simulink model "exampleModel_bus_axi_lcls2"  (R2017b)
settings: Solver=VariableStepAuto  StartTime=0.0  StopTime=10e-5  RelTol=1e-3
PreLoadFcn:
  | setup
values from neighbouring files (symbols this model uses):
  axiClk = 156.25e6    (= 156250000)    [setup.m]    (also in setup_exampleModel_bus_axi_simulink.m; setup_exampleModel_bus_axi_simulink_lcls2.m; setup_lcls2_pcav.m; sysgen_signal.m)
  cav1p1_addr = 204    [setup_exampleModel_bus_axi_simulink.m]    (also in setup_exampleModel_bus_axi_simulink_lcls2.m; setup_lcls2_pcav.m; sysgen_signal.m)
  cav1p2_addr = cav1p1_addr * 2    (= 408)    [setup_exampleModel_bus_axi_simulink.m]    (also in setup_exampleModel_bus_axi_simulink_lcls2.m; setup_lcls2_pcav.m; sysgen_signal.m)
  cav2p1_addr = cav1p1_addr * 3    (= 612)    [setup_exampleModel_bus_axi_simulink.m]    (also in setup_exampleModel_bus_axi_simulink_lcls2.m; setup_lcls2_pcav.m; sysgen_signal.m)
  cav2p2_addr = cav1p1_addr * 4    (= 816)    [setup_exampleModel_bus_axi_simulink.m]    (also in setup_exampleModel_bus_axi_simulink_lcls2.m; setup_lcls2_pcav.m; sysgen_signal.m)
  Fadc = Fs/interleavedChannels    (= 29750000)    [setup.m]    (also in setup_exampleModel_bus_axi_simulink.m = 357000000; setup_exampleModel_bus_axi_simulink_lcls2.m = 351000000; setup_lcls2_pcav.m = 357000000; sysgen_signal.m = 357000000)
  Fproc = 204e6    (= 204000000)    [setup_exampleModel_bus_axi_simulink.m]    (also in setup_exampleModel_bus_axi_simulink_lcls2.m = 200571400; setup_lcls2_pcav.m; sysgen_signal.m)
  Fsig = Fproc/12    (= 17000000)    [setup_exampleModel_bus_axi_simulink.m]    (also in setup_exampleModel_bus_axi_simulink_lcls2.m = 16714283.3333; setup_lcls2_pcav.m)
  Tadc = 1/fadc    (= 2.80112044818e-09)    [cavity_signal.m]    (also in setup_exampleModel_bus_axi_simulink.m; setup_exampleModel_bus_axi_simulink_lcls2.m = 2.849002849e-09; setup_lcls2_pcav.m; setup_pcav_simulink.m)
undefined symbols (not defined in the file or in its folder): AXI4, Lite
libraries: xbsIndex_r4 x2055, llrf_lib x10, simulink x1
(part 10 of 12)

== system exampleModel_bus_axi_lcls2/example/dsp/Cav2/IQ_integration2/IQ_latch_normalize1 ==
  I : Inport
  Q : Inport  Port=2
  Window : Inport  Port=3
  Reset : Inport  Port=4
  Accumulator4 : xbsIndex_r4/Accumulator  operation=Add  n_bits=26  overflow=Wrap  scale=1  rst=on  hasbypass=off  infoeditControl=reset for floating point data type must be asserted for a minimum of 2 cycles  en=off  latency=1  msb_inp=100  msb=100  lsb=-100  use_behavioral_HDL=on  implementation=Fabric  dbl_ovrd=off  block_type=accum
  Accumulator5 : xbsIndex_r4/Accumulator  operation=Add  n_bits=26  overflow=Wrap  scale=1  rst=on  hasbypass=off  infoeditControl=reset for floating point data type must be asserted for a minimum of 2 cycles  en=off  latency=1  msb_inp=100  msb=100  lsb=-100  use_behavioral_HDL=on  implementation=Fabric  dbl_ovrd=off  block_type=accum
  Convert10 : xbsIndex_r4/Convert  gui_display_data_type=Boolean  arith_type=Boolean  n_bits=16  bin_pt=14  float_type=Single  exp_bits=8  fraction_bits=24  quantization=Truncate  overflow=Wrap  en=off  latency=1  pipeline=off  dbl_ovrd=off  block_type=convert
  Convert7 : xbsIndex_r4/Convert  gui_display_data_type=Boolean  arith_type=Boolean  n_bits=16  bin_pt=14  float_type=Single  exp_bits=8  fraction_bits=24  quantization=Truncate  overflow=Wrap  en=off  latency=1  pipeline=off  dbl_ovrd=off  block_type=convert
  Gateway Out{1..2,4..9,11,13..14} (11 alike) : xbsIndex_r4/Gateway Out  inherit_from_input=off  hdl_port=on  rows=1  columns=1  UseAsDAC=off  DACChannel='1'  interface=None  automatic_assignment=on  address_offset=hex2dec('00')  intf_name=''  intf_description=''  timing_constraint=None  locs_specified=off  LOCs={}  io_standard={}  block_type=gatewayout
  Inverter4 : xbsIndex_r4/Inverter  en=off  latency=1  dbl_ovrd=off  block_type=inv
  Inverter5 : xbsIndex_r4/Inverter  en=off  latency=1  dbl_ovrd=off  block_type=inv
  Register3 : xbsIndex_r4/Register  init=0  rst=on  en=on  dbl_ovrd=off  block_type=register
  Register4 : xbsIndex_r4/Register  init=0  rst=on  en=on  dbl_ovrd=off  block_type=register
  Scope1 : Scope  NumInputPorts=4
  Scope2 : Scope  NumInputPorts=4
  Scope4 : Scope  NumInputPorts=4
  Subsystem : Subsystem
  Subsystem4 : Subsystem
  Subsystem5 : Subsystem
  I_out : Outport
  Q_out : Outport  Port=2
  done : Outport  Port=3
  bit : Outport  Port=4
  wires:
  Gateway Out13/1 -> Scope4/3
  Gateway Out11/1 -> Scope4/4
  Gateway Out14/1 -> Scope4/1
  Gateway Out9/1 -> Scope4/2
  Subsystem5/1(q) -> Subsystem/2(Q), Gateway Out14/1
  Subsystem4/1(q) -> Subsystem/1(I), Gateway Out4/1, Gateway Out11/1
  Gateway Out1/1 -> Scope1/2
  Gateway Out7/1 -> Scope2/2
  Gateway Out8/1 -> Scope2/1
  Gateway Out5/1 -> Scope2/4
  Gateway Out6/1 -> Scope2/3
  Accumulator4/1 -> Register3/1, Gateway Out7/1
  Convert7/1 -> Inverter4/1, Register3/3
  Gateway Out4/1 -> Scope1/1
  Gateway Out2/1 -> Scope1/4
  Subsystem/2(Q_norm) -> Q_out/1, Gateway Out9/1
  Subsystem/1(I_norm) -> I_out/1, Gateway Out1/1
  Subsystem/4(bit) -> bit/1, Gateway Out13/1
  Register3/1 -> Subsystem4/1(d)
  Reset/1 -> Register3/2, Register4/2, Subsystem4/2(reset), Gateway Out2/1, Subsystem5/2(reset)
  I/1 -> Accumulator4/1, Gateway Out8/1
  Window/1 -> Convert7/1, Convert10/1
  Register4/1 -> Subsystem5/1(d)
  Subsystem/3(done) -> done/1
  Q/1 -> Accumulator5/1, Gateway Out6/1
  Convert10/1 -> Inverter5/1, Register4/3
  Inverter5/1 -> Accumulator5/2, Subsystem4/3(Latch), Subsystem5/3(Latch)
  Inverter4/1 -> Accumulator4/2
  Accumulator5/1 -> Register4/1, Gateway Out5/1

== system exampleModel_bus_axi_lcls2/example/dsp/Cav2/Subsystem10/posedge_pulse ==
  In1 : Inport
  Inverter1 : xbsIndex_r4/Inverter  en=off  latency=1  dbl_ovrd=off  block_type=inv
  Logical : xbsIndex_r4/Logical  logical_function=AND  inputs=2  en=off  latency=1  precision=Full  arith_type=Unsigned  n_bits=16  bin_pt=0  align_bp=on  dbl_ovrd=off  block_type=logical
  Out1 : Outport
  wires:
  In1/1 -> Logical/1, Inverter1/1
  Logical/1 -> Out1/1
  Inverter1/1 -> Logical/2

== system exampleModel_bus_axi_lcls2/example/dsp/Cav2/Subsystem11/posedge_pulse ==
  In1 : Inport
  Inverter1 : xbsIndex_r4/Inverter  en=off  latency=1  dbl_ovrd=off  block_type=inv
  Logical : xbsIndex_r4/Logical  logical_function=AND  inputs=2  en=off  latency=1  precision=Full  arith_type=Unsigned  n_bits=16  bin_pt=0  align_bp=on  dbl_ovrd=off  block_type=logical
  Out1 : Outport
  wires:
  In1/1 -> Logical/1, Inverter1/1
  Logical/1 -> Out1/1
  Inverter1/1 -> Logical/2

== system exampleModel_bus_axi_lcls2/example/dsp/Cav2/Subsystem12/posedge_pulse ==
  In1 : Inport
  Inverter1 : xbsIndex_r4/Inverter  en=off  latency=1  dbl_ovrd=off  block_type=inv
  Logical : xbsIndex_r4/Logical  logical_function=AND  inputs=2  en=off  latency=1  precision=Full  arith_type=Unsigned  n_bits=16  bin_pt=0  align_bp=on  dbl_ovrd=off  block_type=logical
  Out1 : Outport
  wires:
  Inverter1/1 -> Logical/2
  Logical/1 -> Out1/1
  In1/1 -> Inverter1/1, Logical/1

== system exampleModel_bus_axi_lcls2/example/dsp/Cav2/Subsystem5/posedge_pulse ==
  In1 : Inport
  Inverter1 : xbsIndex_r4/Inverter  en=off  latency=1  dbl_ovrd=off  block_type=inv
  Logical : xbsIndex_r4/Logical  logical_function=AND  inputs=2  en=off  latency=1  precision=Full  arith_type=Unsigned  n_bits=16  bin_pt=0  align_bp=on  dbl_ovrd=off  block_type=logical
  Out1 : Outport
  wires:
  Inverter1/1 -> Logical/2
  Logical/1 -> Out1/1
  In1/1 -> Inverter1/1, Logical/1

== system exampleModel_bus_axi_lcls2/example/dsp/Cav2/Subsystem6/posedge_pulse ==
  In1 : Inport
  Inverter1 : xbsIndex_r4/Inverter  en=off  latency=1  dbl_ovrd=off  block_type=inv
  Logical : xbsIndex_r4/Logical  logical_function=AND  inputs=2  en=off  latency=1  precision=Full  arith_type=Unsigned  n_bits=16  bin_pt=0  align_bp=on  dbl_ovrd=off  block_type=logical
  Out1 : Outport
  wires:
  In1/1 -> Logical/1, Inverter1/1
  Logical/1 -> Out1/1
  Inverter1/1 -> Logical/2

== system exampleModel_bus_axi_lcls2/example/dsp/Cav2/Subsystem7/posedge_pulse ==
  In1 : Inport
  Inverter1 : xbsIndex_r4/Inverter  en=off  latency=1  dbl_ovrd=off  block_type=inv
  Logical : xbsIndex_r4/Logical  logical_function=AND  inputs=2  en=off  latency=1  precision=Full  arith_type=Unsigned  n_bits=16  bin_pt=0  align_bp=on  dbl_ovrd=off  block_type=logical
  Out1 : Outport
  wires:
  Inverter1/1 -> Logical/2
  Logical/1 -> Out1/1
  In1/1 -> Inverter1/1, Logical/1

== system exampleModel_bus_axi_lcls2/example/dsp/Cav2/Subsystem8/posedge_pulse ==
  In1 : Inport
  Inverter1 : xbsIndex_r4/Inverter  en=off  latency=1  dbl_ovrd=off  block_type=inv
  Logical : xbsIndex_r4/Logical  logical_function=AND  inputs=2  en=off  latency=1  precision=Full  arith_type=Unsigned  n_bits=16  bin_pt=0  align_bp=on  dbl_ovrd=off  block_type=logical
  Out1 : Outport
  wires:
  In1/1 -> Logical/1, Inverter1/1
  Logical/1 -> Out1/1
  Inverter1/1 -> Logical/2

== system exampleModel_bus_axi_lcls2/example/dsp/Cav2/Subsystem9/posedge_pulse ==
  In1 : Inport
  Inverter1 : xbsIndex_r4/Inverter  en=off  latency=1  dbl_ovrd=off  block_type=inv
  Logical : xbsIndex_r4/Logical  logical_function=AND  inputs=2  en=off  latency=1  precision=Full  arith_type=Unsigned  n_bits=16  bin_pt=0  align_bp=on  dbl_ovrd=off  block_type=logical
  Out1 : Outport
  wires:
  Inverter1/1 -> Logical/2
  Logical/1 -> Out1/1
  In1/1 -> Inverter1/1, Logical/1

== system exampleModel_bus_axi_lcls2/example/dsp/Cav2/c1p1_PA_conversion/Subsystem1 ==
  d : Inport
  reset : Inport  Port=2
  Latch : Inport  Port=3
  Register11 : xbsIndex_r4/Register  init=0  rst=on  en=on  dbl_ovrd=off  block_type=register
  posedge_pulse : Subsystem
  q : Outport
  wires:
  reset/1 -> Register11/2
  Latch/1 -> posedge_pulse/1(In1)
  posedge_pulse/1(Out1) -> Register11/3
  Register11/1 -> q/1
  d/1 -> Register11/1

== system exampleModel_bus_axi_lcls2/example/dsp/Cav2/c1p1_PA_conversion/Subsystem2 ==
  d : Inport
  reset : Inport  Port=2
  Latch : Inport  Port=3
  Register11 : xbsIndex_r4/Register  init=0  rst=on  en=on  dbl_ovrd=off  block_type=register
  posedge_pulse : Subsystem
  q : Outport
  wires:
  reset/1 -> Register11/2
  Latch/1 -> posedge_pulse/1(In1)
  posedge_pulse/1(Out1) -> Register11/3
  Register11/1 -> q/1
  d/1 -> Register11/1

== system exampleModel_bus_axi_lcls2/example/dsp/Cav2/c1p1_PA_conversion/Subsystem3 ==
  d : Inport
  reset : Inport  Port=2
  Latch : Inport  Port=3
  Register11 : xbsIndex_r4/Register  init=0  rst=on  en=on  dbl_ovrd=off  block_type=register
  posedge_pulse : Subsystem
  q : Outport
  wires:
  d/1 -> Register11/1
  Register11/1 -> q/1
  posedge_pulse/1(Out1) -> Register11/3
  Latch/1 -> posedge_pulse/1(In1)
  reset/1 -> Register11/2

== system exampleModel_bus_axi_lcls2/example/dsp/Cav2/c1p1_PA_conversion/Subsystem4 ==
  d : Inport
  reset : Inport  Port=2
  Latch : Inport  Port=3
  Register11 : xbsIndex_r4/Register  init=0  rst=on  en=on  dbl_ovrd=off  block_type=register
  posedge_pulse : Subsystem
  q : Outport
  wires:
  d/1 -> Register11/1
  Register11/1 -> q/1
  posedge_pulse/1(Out1) -> Register11/3
  Latch/1 -> posedge_pulse/1(In1)
  reset/1 -> Register11/2

== system exampleModel_bus_axi_lcls2/example/dsp/Cav2/c1p1_PA_conversion1/Subsystem1 ==
  d : Inport
  reset : Inport  Port=2
  Latch : Inport  Port=3
  Register11 : xbsIndex_r4/Register  init=0  rst=on  en=on  dbl_ovrd=off  block_type=register
  posedge_pulse : Subsystem
  q : Outport
  wires:
  reset/1 -> Register11/2
  Latch/1 -> posedge_pulse/1(In1)
  posedge_pulse/1(Out1) -> Register11/3
  Register11/1 -> q/1
  d/1 -> Register11/1

== system exampleModel_bus_axi_lcls2/example/dsp/Cav2/c1p1_PA_conversion1/Subsystem2 ==
  d : Inport
  reset : Inport  Port=2
  Latch : Inport  Port=3
  Register11 : xbsIndex_r4/Register  init=0  rst=on  en=on  dbl_ovrd=off  block_type=register
  posedge_pulse : Subsystem
  q : Outport
  wires:
  reset/1 -> Register11/2
  Latch/1 -> posedge_pulse/1(In1)
  posedge_pulse/1(Out1) -> Register11/3
  Register11/1 -> q/1
  d/1 -> Register11/1

== system exampleModel_bus_axi_lcls2/example/dsp/Cav2/c1p1_PA_conversion1/Subsystem3 ==
  d : Inport
  reset : Inport  Port=2
  Latch : Inport  Port=3
  Register11 : xbsIndex_r4/Register  init=0  rst=on  en=on  dbl_ovrd=off  block_type=register
  posedge_pulse : Subsystem
  q : Outport
  wires:
  d/1 -> Register11/1
  Register11/1 -> q/1
  posedge_pulse/1(Out1) -> Register11/3
  Latch/1 -> posedge_pulse/1(In1)
  reset/1 -> Register11/2

== system exampleModel_bus_axi_lcls2/example/dsp/Cav2/c1p1_PA_conversion1/Subsystem4 ==
  d : Inport
  reset : Inport  Port=2
  Latch : Inport  Port=3
  Register11 : xbsIndex_r4/Register  init=0  rst=on  en=on  dbl_ovrd=off  block_type=register
  posedge_pulse : Subsystem
  q : Outport
  wires:
  d/1 -> Register11/1
  Register11/1 -> q/1
  posedge_pulse/1(Out1) -> Register11/3
  Latch/1 -> posedge_pulse/1(In1)
  reset/1 -> Register11/2

== system exampleModel_bus_axi_lcls2/example/dsp/Cav2/c1p2_freq_err_module1/freq_err1 ==
  note: find ratio with NCO
  note: 2*pi*dt
  note: w = d_phi/dt
  note: f=w/(2*pi)
  note: window for start/stop evaluating the phase
  raw_phase : Inport
  window : Inport  Port=2
  reset : Inport  Port=3
  Constant8 : xbsIndex_r4/Constant  const=-Fsig  gui_display_data_type=Fixed-point  arith_type=Signed (2's comp)  n_bits=26  bin_pt=0  preci_type=Single  exp_width=8  frac_width=24  explicit_period=off  period=1  equ=P=C  opselect=C  inp2=PCIN>>17  opr=+  inp1=P  carry=CIN  dbl_ovrd=off  block_type=constant
  Convert : xbsIndex_r4/Convert  gui_display_data_type=Fixed-point  arith_type="Signed  (2's comp)"  n_bits=32  bin_pt=32  float_type=Single  exp_bits=8  fraction_bits=24  quantization=Truncate  overflow=Saturate  en=off  latency=1  pipeline=off  dbl_ovrd=off  block_type=convert
  Convert1 : xbsIndex_r4/Convert  gui_display_data_type=Fixed-point  arith_type="Signed  (2's comp)"  n_bits=32  bin_pt=18  float_type=Single  exp_bits=8  fraction_bits=24  quantization=Truncate  overflow=Saturate  en=off  latency=1  pipeline=off  dbl_ovrd=off  block_type=convert
  Convert3 : xbsIndex_r4/Convert  gui_display_data_type=Boolean  arith_type=Boolean  n_bits=16  bin_pt=14  float_type=Single  exp_bits=8  fraction_bits=24  quantization=Truncate  overflow=Wrap  en=off  latency=1  pipeline=off  dbl_ovrd=off  block_type=convert
  Delay1 : xbsIndex_r4/Delay  rst=off  infoeditControl=Selection of Reset will increase slice count due to use of real FFs and instead of SRLs  en=off  latency=3  reg_retiming=off  dbl_ovrd=off  block_type=delay
  Delay2 : xbsIndex_r4/Delay  rst=off  infoeditControl=Selection of Reset will increase slice count due to use of real FFs and instead of SRLs  en=off  latency=3  reg_retiming=off  dbl_ovrd=off  block_type=delay
  Delay3 : xbsIndex_r4/Delay  rst=off  infoeditControl=Selection of Reset will increase slice count due to use of real FFs and instead of SRLs  en=off  latency=3  reg_retiming=off  dbl_ovrd=off  block_type=delay
  Display6 : Display
  Display8 : Display
  Divide : xbsIndex_r4/Divide  flow_control=NonBlocking  axi_optimize_goal=Resources  algorithm_type=Radix2  infoedit1=Specify output fraction-width for Fixed-point division.  fractional_width=32  infoedit2=Specify latency for Floating-point division.  latency=1  rate=1  has_a_tlast=off  has_a_tuser=off  has_b_tlast=off  has_b_tuser=off  en=off  has_result_tready=off  result_tlast_behv=Pass_A_TLAST  has_underflow=off  has_overflow=off  has_invalid_op=off  has_divide_by_zero=off  fpo_op_type=mergeddivide  block_type=divide
      settings: infoedit=Blocking: Wait for data on all inputs, allow back-pressure.<br>NonBlocking: operate every cycle in which all inputs are valid, no back-pressure.
  Divide1 : xbsIndex_r4/Divide  flow_control=NonBlocking  axi_optimize_goal=Resources  algorithm_type=Radix2  infoedit1=Specify output fraction-width for Fixed-point division.  fractional_width=33  infoedit2=Specify latency for Floating-point division.  latency=1  rate=1  has_a_tlast=off  has_a_tuser=off  has_b_tlast=off  has_b_tuser=off  en=off  has_result_tready=off  result_tlast_behv=Pass_A_TLAST  has_underflow=off  has_overflow=off  has_invalid_op=off  has_divide_by_zero=off  fpo_op_type=mergeddivide  block_type=divide
      settings: infoedit=Blocking: Wait for data on all inputs, allow back-pressure.<br>NonBlocking: operate every cycle in which all inputs are valid, no back-pressure.
  Down Sample : xbsIndex_r4/Down Sample  sample_ratio=12  sample_phase="Last Value of Frame  (most efficient)"  en=off  rst=off  latency=1  dbl_ovrd=off  block_type=dsamp
  Down Sample2 : xbsIndex_r4/Down Sample  sample_ratio=12  sample_phase="Last Value of Frame  (most efficient)"  en=off  rst=off  latency=1  dbl_ovrd=off  block_type=dsamp
  Gateway Out1 : xbsIndex_r4/Gateway Out  Commented=on  inherit_from_input=off  hdl_port=on  rows=1  columns=1  UseAsDAC=off  DACChannel='1'  interface=None  automatic_assignment=on  address_offset=hex2dec('00')  intf_name=''  intf_description=''  timing_constraint=None  locs_specified=off  LOCs={}  io_standard={}  block_type=gatewayout
  Gateway Out{3..5,11,19..20} (6 alike) : xbsIndex_r4/Gateway Out  inherit_from_input=off  hdl_port=on  rows=1  columns=1  UseAsDAC=off  DACChannel='1'  interface=None  automatic_assignment=on  address_offset=hex2dec('00')  intf_name=''  intf_description=''  timing_constraint=None  locs_specified=off  LOCs={}  io_standard={}  block_type=gatewayout
  Gateway Out6 : xbsIndex_r4/Gateway Out  Commented=on  inherit_from_input=off  hdl_port=on  rows=1  columns=1  UseAsDAC=off  DACChannel='1'  interface=None  automatic_assignment=on  address_offset=hex2dec('00')  intf_name=''  intf_description=''  timing_constraint=None  locs_specified=off  LOCs={}  io_standard={}  block_type=gatewayout
  Mult3 : xbsIndex_r4/Mult  precision=User Defined  arith_type="Signed  (2's comp)"  n_bits=18  bin_pt=15  quantization=Truncate  overflow=Saturate  en=off  latency=3  use_behavioral_HDL=off  opt=Speed  use_embedded=on  optimum_pipeline=off  pipeline=on  dbl_ovrd=off  use_rpm=on  placement_style=Triangular  block_type=mult
  Register2 : xbsIndex_r4/Register  init=0  rst=on  en=on  dbl_ovrd=off  block_type=register
  Scope2 : Scope  NumInputPorts=3
  Scope3 : Scope  Commented=on  NumInputPorts=3
  delta_phi : Subsystem
  delta_t : Subsystem
  lo_bit_phi : Scope  NumInputPorts=4
  negedge_pulse : Subsystem  Commented=on
  posedge_pulse : Subsystem  Commented=on
  NCO_err : Outport
  freq_err : Outport  Port=2
  tag scope: cav2_freq_phase_windowed=global
  wires:
  delta_t/1(dt) -> Divide/2
  delta_phi/1(d_phi) -> Divide/1
  Down Sample2/1 -> Gateway Out5/1, freq_err/1
  window/1 -> Delay1/1, Mult3/1, delta_t/1(window), delta_phi/2(window)
  Delay3/1 -> Gateway Out4/1
  Delay2/1 -> Gateway Out3/1
  Delay1/1 -> Gateway Out20/1, negedge_pulse/1(In1), posedge_pulse/1(In1)
  Gateway Out1/1 -> Scope3/3
  posedge_pulse/1(Out1) -> Gateway Out1/1
  negedge_pulse/1(Out1) -> Gateway Out6/1
  Gateway Out6/1 -> Scope3/1
  Register2/1 -> Convert1/1, Divide1/1
  delta_phi/2(val_latched) -> Register2/3
  reset/1 -> Convert3/1
  Gateway Out11/1 -> Scope2/2, Display8/1
  Gateway Out5/1 -> Display6/1, Scope2/1
  Convert3/1 -> delta_t/2(reset), Register2/2, delta_phi/3(reset)
  Gateway Out19/1 -> lo_bit_phi/2
  Mult3/1 -> [cav2_freq_phase_windowed], delta_phi/1(phase), Gateway Out19/1
  Constant8/1 -> Divide1/2
  Down Sample/1 -> Convert/1
  Divide1/1 -> Down Sample/1
  Gateway Out3/1 -> lo_bit_phi/3
  [cav1_pt_cntr] -> Delay3/1
  Gateway Out4/1 -> lo_bit_phi/4
  raw_phase/1 -> Mult3/2, Delay2/1
  Gateway Out20/1 -> Scope3/2, Scope2/3, lo_bit_phi/1
  Convert/1 -> NCO_err/1, Gateway Out11/1
  Divide/1 -> Register2/1
  Convert1/1 -> Down Sample2/1

== system exampleModel_bus_axi_lcls2/example/dsp/Cav2/c1p2_freq_err_module2/freq_err1 ==
  note: find ratio with NCO
  note: 2*pi*dt
  note: w = d_phi/dt
  note: f=w/(2*pi)
  note: window for start/stop evaluating the phase
  raw_phase : Inport
  window : Inport  Port=2
  reset : Inport  Port=3
  Constant8 : xbsIndex_r4/Constant  const=-Fsig  gui_display_data_type=Fixed-point  arith_type=Signed (2's comp)  n_bits=26  bin_pt=0  preci_type=Single  exp_width=8  frac_width=24  explicit_period=off  period=1  equ=P=C  opselect=C  inp2=PCIN>>17  opr=+  inp1=P  carry=CIN  dbl_ovrd=off  block_type=constant
  Convert : xbsIndex_r4/Convert  gui_display_data_type=Fixed-point  arith_type="Signed  (2's comp)"  n_bits=32  bin_pt=32  float_type=Single  exp_bits=8  fraction_bits=24  quantization=Truncate  overflow=Saturate  en=off  latency=1  pipeline=off  dbl_ovrd=off  block_type=convert
  Convert1 : xbsIndex_r4/Convert  gui_display_data_type=Fixed-point  arith_type="Signed  (2's comp)"  n_bits=32  bin_pt=18  float_type=Single  exp_bits=8  fraction_bits=24  quantization=Truncate  overflow=Saturate  en=off  latency=1  pipeline=off  dbl_ovrd=off  block_type=convert
  Convert3 : xbsIndex_r4/Convert  gui_display_data_type=Boolean  arith_type=Boolean  n_bits=16  bin_pt=14  float_type=Single  exp_bits=8  fraction_bits=24  quantization=Truncate  overflow=Wrap  en=off  latency=1  pipeline=off  dbl_ovrd=off  block_type=convert
  Delay1 : xbsIndex_r4/Delay  rst=off  infoeditControl=Selection of Reset will increase slice count due to use of real FFs and instead of SRLs  en=off  latency=3  reg_retiming=off  dbl_ovrd=off  block_type=delay
  Delay2 : xbsIndex_r4/Delay  rst=off  infoeditControl=Selection of Reset will increase slice count due to use of real FFs and instead of SRLs  en=off  latency=3  reg_retiming=off  dbl_ovrd=off  block_type=delay
  Delay3 : xbsIndex_r4/Delay  rst=off  infoeditControl=Selection of Reset will increase slice count due to use of real FFs and instead of SRLs  en=off  latency=3  reg_retiming=off  dbl_ovrd=off  block_type=delay
  Display6 : Display
  Display8 : Display
  Divide : xbsIndex_r4/Divide  flow_control=NonBlocking  axi_optimize_goal=Resources  algorithm_type=Radix2  infoedit1=Specify output fraction-width for Fixed-point division.  fractional_width=32  infoedit2=Specify latency for Floating-point division.  latency=1  rate=1  has_a_tlast=off  has_a_tuser=off  has_b_tlast=off  has_b_tuser=off  en=off  has_result_tready=off  result_tlast_behv=Pass_A_TLAST  has_underflow=off  has_overflow=off  has_invalid_op=off  has_divide_by_zero=off  fpo_op_type=mergeddivide  block_type=divide
      settings: infoedit=Blocking: Wait for data on all inputs, allow back-pressure.<br>NonBlocking: operate every cycle in which all inputs are valid, no back-pressure.
  Divide1 : xbsIndex_r4/Divide  flow_control=NonBlocking  axi_optimize_goal=Resources  algorithm_type=Radix2  infoedit1=Specify output fraction-width for Fixed-point division.  fractional_width=33  infoedit2=Specify latency for Floating-point division.  latency=1  rate=1  has_a_tlast=off  has_a_tuser=off  has_b_tlast=off  has_b_tuser=off  en=off  has_result_tready=off  result_tlast_behv=Pass_A_TLAST  has_underflow=off  has_overflow=off  has_invalid_op=off  has_divide_by_zero=off  fpo_op_type=mergeddivide  block_type=divide
      settings: infoedit=Blocking: Wait for data on all inputs, allow back-pressure.<br>NonBlocking: operate every cycle in which all inputs are valid, no back-pressure.
  Down Sample : xbsIndex_r4/Down Sample  sample_ratio=12  sample_phase="Last Value of Frame  (most efficient)"  en=off  rst=off  latency=1  dbl_ovrd=off  block_type=dsamp
  Down Sample2 : xbsIndex_r4/Down Sample  sample_ratio=12  sample_phase="Last Value of Frame  (most efficient)"  en=off  rst=off  latency=1  dbl_ovrd=off  block_type=dsamp
  Gateway Out1 : xbsIndex_r4/Gateway Out  Commented=on  inherit_from_input=off  hdl_port=on  rows=1  columns=1  UseAsDAC=off  DACChannel='1'  interface=None  automatic_assignment=on  address_offset=hex2dec('00')  intf_name=''  intf_description=''  timing_constraint=None  locs_specified=off  LOCs={}  io_standard={}  block_type=gatewayout
  Gateway Out{3..5,11,19..20} (6 alike) : xbsIndex_r4/Gateway Out  inherit_from_input=off  hdl_port=on  rows=1  columns=1  UseAsDAC=off  DACChannel='1'  interface=None  automatic_assignment=on  address_offset=hex2dec('00')  intf_name=''  intf_description=''  timing_constraint=None  locs_specified=off  LOCs={}  io_standard={}  block_type=gatewayout
  Gateway Out6 : xbsIndex_r4/Gateway Out  Commented=on  inherit_from_input=off  hdl_port=on  rows=1  columns=1  UseAsDAC=off  DACChannel='1'  interface=None  automatic_assignment=on  address_offset=hex2dec('00')  intf_name=''  intf_description=''  timing_constraint=None  locs_specified=off  LOCs={}  io_standard={}  block_type=gatewayout
  Mult3 : xbsIndex_r4/Mult  precision=User Defined  arith_type="Signed  (2's comp)"  n_bits=18  bin_pt=15  quantization=Truncate  overflow=Saturate  en=off  latency=3  use_behavioral_HDL=off  opt=Speed  use_embedded=on  optimum_pipeline=off  pipeline=on  dbl_ovrd=off  use_rpm=on  placement_style=Triangular  block_type=mult
  Register2 : xbsIndex_r4/Register  init=0  rst=on  en=on  dbl_ovrd=off  block_type=register
  Scope2 : Scope  NumInputPorts=3
  Scope3 : Scope  Commented=on  NumInputPorts=3
  delta_phi : Subsystem
  delta_t : Subsystem
  lo_bit_phi : Scope  NumInputPorts=4
  negedge_pulse : Subsystem  Commented=on
  posedge_pulse : Subsystem  Commented=on
  NCO_err : Outport
  freq_err : Outport  Port=2
  wires:
  delta_t/1(dt) -> Divide/2
  delta_phi/1(d_phi) -> Divide/1
  Down Sample2/1 -> Gateway Out5/1, freq_err/1
  window/1 -> Delay1/1, Mult3/1, delta_t/1(window), delta_phi/2(window)
  Delay3/1 -> Gateway Out4/1
  Delay2/1 -> Gateway Out3/1
  Delay1/1 -> Gateway Out20/1, negedge_pulse/1(In1), posedge_pulse/1(In1)
  Gateway Out1/1 -> Scope3/3
  posedge_pulse/1(Out1) -> Gateway Out1/1
  negedge_pulse/1(Out1) -> Gateway Out6/1
  Gateway Out6/1 -> Scope3/1
  Register2/1 -> Convert1/1, Divide1/1
  delta_phi/2(val_latched) -> Register2/3
  reset/1 -> Convert3/1
  Gateway Out11/1 -> Scope2/2, Display8/1
  Gateway Out5/1 -> Display6/1, Scope2/1
  Convert3/1 -> delta_t/2(reset), Register2/2, delta_phi/3(reset)
  Gateway Out19/1 -> lo_bit_phi/2
  Mult3/1 -> delta_phi/1(phase), Gateway Out19/1
  Constant8/1 -> Divide1/2
  Down Sample/1 -> Convert/1
  Divide1/1 -> Down Sample/1
  Gateway Out3/1 -> lo_bit_phi/3
  [cav1_pt_cntr] -> Delay3/1
  Gateway Out4/1 -> lo_bit_phi/4
  raw_phase/1 -> Mult3/2, Delay2/1
  Gateway Out20/1 -> Scope3/2, Scope2/3, lo_bit_phi/1
  Convert/1 -> NCO_err/1, Gateway Out11/1
  Divide/1 -> Register2/1
  Convert1/1 -> Down Sample2/1

== system exampleModel_bus_axi_lcls2/example/dsp/Cav1/IQ_integration1/IQ_latch_normalize/Subsystem ==
  I : Inport
  Q : Inport  Port=2
  Absolute : xbsIndex_r4/Absolute  precision=Full  arith_type=Unsigned  n_bits=16  bin_pt=14  quantization=Truncate  overflow=Wrap  en=off  latency=1  dbl_ovrd=off  block_type=abs
  Absolute1 : xbsIndex_r4/Absolute  precision=Full  arith_type=Unsigned  n_bits=16  bin_pt=14  quantization=Truncate  overflow=Wrap  en=off  latency=1  dbl_ovrd=off  block_type=abs
  Convert4 : xbsIndex_r4/Convert  gui_display_data_type=Fixed-point  arith_type="Signed  (2's comp)"  n_bits=18  bin_pt=16  float_type=Single  exp_bits=8  fraction_bits=24  quantization=Truncate  overflow=Wrap  en=off  latency=1  pipeline=off  dbl_ovrd=off  block_type=convert
  Convert9 : xbsIndex_r4/Convert  gui_display_data_type=Fixed-point  arith_type="Signed  (2's comp)"  n_bits=18  bin_pt=16  float_type=Single  exp_bits=8  fraction_bits=24  quantization=Truncate  overflow=Wrap  en=off  latency=1  pipeline=off  dbl_ovrd=off  block_type=convert
  Delay : xbsIndex_r4/Delay  rst=off  infoeditControl=Selection of Reset will increase slice count due to use of real FFs and instead of SRLs  en=off  latency=1  reg_retiming=off  dbl_ovrd=off  block_type=delay
  Delay1 : xbsIndex_r4/Delay  rst=off  infoeditControl=Selection of Reset will increase slice count due to use of real FFs and instead of SRLs  en=off  latency=1  reg_retiming=off  dbl_ovrd=off  block_type=delay
  Display2 : Display
  Gateway Out{1..6,22,24,27} (9 alike) : xbsIndex_r4/Gateway Out  inherit_from_input=off  hdl_port=on  rows=1  columns=1  UseAsDAC=off  DACChannel='1'  interface=None  automatic_assignment=on  address_offset=hex2dec('00')  intf_name=''  intf_description=''  timing_constraint=None  locs_specified=off  LOCs={}  io_standard={}  block_type=gatewayout
  MCode : xbsIndex_r4/MCode  mfname=integration_normalize  explicit_period=off  period=1  inputsTable={'boundInpExpr'=>['','','',''],'inputs'=>['I_int','Q_int','I_int_abs','Q_int_abs']}  outputsTable={'outputs'=>['I_norm','Q_norm','done','bit'],'suppressOut'=>['off','off','off','off']}  enable_stdout=off  enable_debug=off  suppress_output=on  defparams={}  hide_port_list={}  dbl_ovrd=off  block_type=mcode
  Scope1 : Scope  NumInputPorts=4
  Scope11 : Scope  NumInputPorts=4
  I_norm : Outport
  Q_norm : Outport  Port=2
  done : Outport  Port=3
  bit : Outport  Port=4
  wires:
  MCode/3 -> done/1
  Absolute1/1 -> MCode/4
  Gateway Out22/1 -> Scope11/2
  Delay1/1 -> Gateway Out6/1, MCode/2
  Q/1 -> Delay1/1, Absolute1/1
  Absolute/1 -> MCode/3
  MCode/4 -> bit/1, Gateway Out27/1
  I/1 -> Absolute/1, Delay/1
  MCode/2 -> Gateway Out5/1, Gateway Out4/1, Convert4/1
  Gateway Out24/1 -> Scope11/1
  Gateway Out27/1 -> Display2/1
  Delay/1 -> Gateway Out24/1, MCode/1
  MCode/1 -> Gateway Out3/1, Convert9/1, Gateway Out22/1
  Convert4/1 -> Q_norm/1, Gateway Out1/1
  Convert9/1 -> I_norm/1, Gateway Out2/1
  Gateway Out1/1 -> Scope1/2
  Gateway Out2/1 -> Scope1/4
  Gateway Out4/1 -> Scope1/1
  Gateway Out3/1 -> Scope1/3
  Gateway Out6/1 -> Scope11/3
  Gateway Out5/1 -> Scope11/4

== system exampleModel_bus_axi_lcls2/example/dsp/Cav1/IQ_integration1/IQ_latch_normalize/Subsystem4 ==
  d : Inport
  reset : Inport  Port=2
  Latch : Inport  Port=3
  Register11 : xbsIndex_r4/Register  init=0  rst=on  en=on  dbl_ovrd=off  block_type=register
  posedge_pulse : Subsystem
  q : Outport
  wires:
  d/1 -> Register11/1
  Register11/1 -> q/1
  posedge_pulse/1(Out1) -> Register11/3
  Latch/1 -> posedge_pulse/1(In1)
  reset/1 -> Register11/2

== system exampleModel_bus_axi_lcls2/example/dsp/Cav1/IQ_integration1/IQ_latch_normalize/Subsystem5 ==
  d : Inport
  reset : Inport  Port=2
  Latch : Inport  Port=3
  Register11 : xbsIndex_r4/Register  init=0  rst=on  en=on  dbl_ovrd=off  block_type=register
  posedge_pulse : Subsystem
  q : Outport
  wires:
  reset/1 -> Register11/2
  Latch/1 -> posedge_pulse/1(In1)
  posedge_pulse/1(Out1) -> Register11/3
  Register11/1 -> q/1
  d/1 -> Register11/1

== system exampleModel_bus_axi_lcls2/example/dsp/Cav1/IQ_integration1/IQ_latch_normalize1/Subsystem ==
  I : Inport
  Q : Inport  Port=2
  Absolute : xbsIndex_r4/Absolute  precision=Full  arith_type=Unsigned  n_bits=16  bin_pt=14  quantization=Truncate  overflow=Wrap  en=off  latency=1  dbl_ovrd=off  block_type=abs
  Absolute1 : xbsIndex_r4/Absolute  precision=Full  arith_type=Unsigned  n_bits=16  bin_pt=14  quantization=Truncate  overflow=Wrap  en=off  latency=1  dbl_ovrd=off  block_type=abs
  Convert4 : xbsIndex_r4/Convert  gui_display_data_type=Fixed-point  arith_type="Signed  (2's comp)"  n_bits=18  bin_pt=16  float_type=Single  exp_bits=8  fraction_bits=24  quantization=Truncate  overflow=Wrap  en=off  latency=1  pipeline=off  dbl_ovrd=off  block_type=convert
  Convert9 : xbsIndex_r4/Convert  gui_display_data_type=Fixed-point  arith_type="Signed  (2's comp)"  n_bits=18  bin_pt=16  float_type=Single  exp_bits=8  fraction_bits=24  quantization=Truncate  overflow=Wrap  en=off  latency=1  pipeline=off  dbl_ovrd=off  block_type=convert
  Delay : xbsIndex_r4/Delay  rst=off  infoeditControl=Selection of Reset will increase slice count due to use of real FFs and instead of SRLs  en=off  latency=1  reg_retiming=off  dbl_ovrd=off  block_type=delay
  Delay1 : xbsIndex_r4/Delay  rst=off  infoeditControl=Selection of Reset will increase slice count due to use of real FFs and instead of SRLs  en=off  latency=1  reg_retiming=off  dbl_ovrd=off  block_type=delay
  Display2 : Display
  Gateway Out{1..6,22,24,27} (9 alike) : xbsIndex_r4/Gateway Out  inherit_from_input=off  hdl_port=on  rows=1  columns=1  UseAsDAC=off  DACChannel='1'  interface=None  automatic_assignment=on  address_offset=hex2dec('00')  intf_name=''  intf_description=''  timing_constraint=None  locs_specified=off  LOCs={}  io_standard={}  block_type=gatewayout
  MCode : xbsIndex_r4/MCode  mfname=integration_normalize  explicit_period=off  period=1  inputsTable={'boundInpExpr'=>['','','',''],'inputs'=>['I_int','Q_int','I_int_abs','Q_int_abs']}  outputsTable={'outputs'=>['I_norm','Q_norm','done','bit'],'suppressOut'=>['off','off','off','off']}  enable_stdout=off  enable_debug=off  suppress_output=on  defparams={}  hide_port_list={}  dbl_ovrd=off  block_type=mcode
  Scope1 : Scope  NumInputPorts=4
  Scope11 : Scope  NumInputPorts=4
  I_norm : Outport
  Q_norm : Outport  Port=2
  done : Outport  Port=3
  bit : Outport  Port=4
  wires:
  Gateway Out5/1 -> Scope11/4
  Gateway Out6/1 -> Scope11/3
  Gateway Out3/1 -> Scope1/3
  Gateway Out4/1 -> Scope1/1
  Gateway Out2/1 -> Scope1/4
  Gateway Out1/1 -> Scope1/2
  Convert9/1 -> Gateway Out2/1, I_norm/1
  Convert4/1 -> Gateway Out1/1, Q_norm/1
  MCode/1 -> Gateway Out22/1, Convert9/1, Gateway Out3/1
  Delay/1 -> MCode/1, Gateway Out24/1
  Gateway Out27/1 -> Display2/1
  Gateway Out24/1 -> Scope11/1
  MCode/2 -> Convert4/1, Gateway Out4/1, Gateway Out5/1
  I/1 -> Delay/1, Absolute/1
  MCode/4 -> Gateway Out27/1, bit/1
  Absolute/1 -> MCode/3
  Q/1 -> Absolute1/1, Delay1/1
  Delay1/1 -> MCode/2, Gateway Out6/1
  Gateway Out22/1 -> Scope11/2
  Absolute1/1 -> MCode/4
  MCode/3 -> done/1

== system exampleModel_bus_axi_lcls2/example/dsp/Cav1/IQ_integration1/IQ_latch_normalize1/Subsystem4 ==
  d : Inport
  reset : Inport  Port=2
  Latch : Inport  Port=3
  Register11 : xbsIndex_r4/Register  init=0  rst=on  en=on  dbl_ovrd=off  block_type=register
  posedge_pulse : Subsystem
  q : Outport
  wires:
  reset/1 -> Register11/2
  Latch/1 -> posedge_pulse/1(In1)
  posedge_pulse/1(Out1) -> Register11/3
  Register11/1 -> q/1
  d/1 -> Register11/1

== system exampleModel_bus_axi_lcls2/example/dsp/Cav1/IQ_integration1/IQ_latch_normalize1/Subsystem5 ==
  d : Inport
  reset : Inport  Port=2
  Latch : Inport  Port=3
  Register11 : xbsIndex_r4/Register  init=0  rst=on  en=on  dbl_ovrd=off  block_type=register
  posedge_pulse : Subsystem
  q : Outport
  wires:
  d/1 -> Register11/1
  Register11/1 -> q/1
  posedge_pulse/1(Out1) -> Register11/3
  Latch/1 -> posedge_pulse/1(In1)
  reset/1 -> Register11/2

== system exampleModel_bus_axi_lcls2/example/dsp/Cav1/IQ_integration2/IQ_latch_normalize/Subsystem ==
  I : Inport
  Q : Inport  Port=2
  Absolute : xbsIndex_r4/Absolute  precision=Full  arith_type=Unsigned  n_bits=16  bin_pt=14  quantization=Truncate  overflow=Wrap  en=off  latency=1  dbl_ovrd=off  block_type=abs
  Absolute1 : xbsIndex_r4/Absolute  precision=Full  arith_type=Unsigned  n_bits=16  bin_pt=14  quantization=Truncate  overflow=Wrap  en=off  latency=1  dbl_ovrd=off  block_type=abs
  Convert4 : xbsIndex_r4/Convert  gui_display_data_type=Fixed-point  arith_type="Signed  (2's comp)"  n_bits=18  bin_pt=16  float_type=Single  exp_bits=8  fraction_bits=24  quantization=Truncate  overflow=Wrap  en=off  latency=1  pipeline=off  dbl_ovrd=off  block_type=convert
  Convert9 : xbsIndex_r4/Convert  gui_display_data_type=Fixed-point  arith_type="Signed  (2's comp)"  n_bits=18  bin_pt=16  float_type=Single  exp_bits=8  fraction_bits=24  quantization=Truncate  overflow=Wrap  en=off  latency=1  pipeline=off  dbl_ovrd=off  block_type=convert
  Delay : xbsIndex_r4/Delay  rst=off  infoeditControl=Selection of Reset will increase slice count due to use of real FFs and instead of SRLs  en=off  latency=1  reg_retiming=off  dbl_ovrd=off  block_type=delay
  Delay1 : xbsIndex_r4/Delay  rst=off  infoeditControl=Selection of Reset will increase slice count due to use of real FFs and instead of SRLs  en=off  latency=1  reg_retiming=off  dbl_ovrd=off  block_type=delay
  Display2 : Display
  Gateway Out{1..6,22,24,27} (9 alike) : xbsIndex_r4/Gateway Out  inherit_from_input=off  hdl_port=on  rows=1  columns=1  UseAsDAC=off  DACChannel='1'  interface=None  automatic_assignment=on  address_offset=hex2dec('00')  intf_name=''  intf_description=''  timing_constraint=None  locs_specified=off  LOCs={}  io_standard={}  block_type=gatewayout
  MCode : xbsIndex_r4/MCode  mfname=integration_normalize  explicit_period=off  period=1  inputsTable={'boundInpExpr'=>['','','',''],'inputs'=>['I_int','Q_int','I_int_abs','Q_int_abs']}  outputsTable={'outputs'=>['I_norm','Q_norm','done','bit'],'suppressOut'=>['off','off','off','off']}  enable_stdout=off  enable_debug=off  suppress_output=on  defparams={}  hide_port_list={}  dbl_ovrd=off  block_type=mcode
  Scope1 : Scope  NumInputPorts=4
  Scope11 : Scope  NumInputPorts=4
  I_norm : Outport
  Q_norm : Outport  Port=2
  done : Outport  Port=3
  bit : Outport  Port=4
  wires:
  MCode/3 -> done/1
  Absolute1/1 -> MCode/4
  Gateway Out22/1 -> Scope11/2
  Delay1/1 -> Gateway Out6/1, MCode/2
  Q/1 -> Delay1/1, Absolute1/1
  Absolute/1 -> MCode/3
  MCode/4 -> bit/1, Gateway Out27/1
  I/1 -> Absolute/1, Delay/1
  MCode/2 -> Gateway Out5/1, Gateway Out4/1, Convert4/1
  Gateway Out24/1 -> Scope11/1
  Gateway Out27/1 -> Display2/1
  Delay/1 -> Gateway Out24/1, MCode/1
  MCode/1 -> Gateway Out3/1, Convert9/1, Gateway Out22/1
  Convert4/1 -> Q_norm/1, Gateway Out1/1
  Convert9/1 -> I_norm/1, Gateway Out2/1
  Gateway Out1/1 -> Scope1/2
  Gateway Out2/1 -> Scope1/4
  Gateway Out4/1 -> Scope1/1
  Gateway Out3/1 -> Scope1/3
  Gateway Out6/1 -> Scope11/3
  Gateway Out5/1 -> Scope11/4

== system exampleModel_bus_axi_lcls2/example/dsp/Cav1/IQ_integration2/IQ_latch_normalize/Subsystem4 ==
  d : Inport
  reset : Inport  Port=2
  Latch : Inport  Port=3
  Register11 : xbsIndex_r4/Register  init=0  rst=on  en=on  dbl_ovrd=off  block_type=register
  posedge_pulse : Subsystem
  q : Outport
  wires:
  d/1 -> Register11/1
  Register11/1 -> q/1
  posedge_pulse/1(Out1) -> Register11/3
  Latch/1 -> posedge_pulse/1(In1)
  reset/1 -> Register11/2

== system exampleModel_bus_axi_lcls2/example/dsp/Cav1/IQ_integration2/IQ_latch_normalize/Subsystem5 ==
  d : Inport
  reset : Inport  Port=2
  Latch : Inport  Port=3
  Register11 : xbsIndex_r4/Register  init=0  rst=on  en=on  dbl_ovrd=off  block_type=register
  posedge_pulse : Subsystem
  q : Outport
  wires:
  reset/1 -> Register11/2
  Latch/1 -> posedge_pulse/1(In1)
  posedge_pulse/1(Out1) -> Register11/3
  Register11/1 -> q/1
  d/1 -> Register11/1

== system exampleModel_bus_axi_lcls2/example/dsp/Cav1/IQ_integration2/IQ_latch_normalize1/Subsystem ==
  I : Inport
  Q : Inport  Port=2
  Absolute : xbsIndex_r4/Absolute  precision=Full  arith_type=Unsigned  n_bits=16  bin_pt=14  quantization=Truncate  overflow=Wrap  en=off  latency=1  dbl_ovrd=off  block_type=abs
  Absolute1 : xbsIndex_r4/Absolute  precision=Full  arith_type=Unsigned  n_bits=16  bin_pt=14  quantization=Truncate  overflow=Wrap  en=off  latency=1  dbl_ovrd=off  block_type=abs
  Convert4 : xbsIndex_r4/Convert  gui_display_data_type=Fixed-point  arith_type="Signed  (2's comp)"  n_bits=18  bin_pt=16  float_type=Single  exp_bits=8  fraction_bits=24  quantization=Truncate  overflow=Wrap  en=off  latency=1  pipeline=off  dbl_ovrd=off  block_type=convert
  Convert9 : xbsIndex_r4/Convert  gui_display_data_type=Fixed-point  arith_type="Signed  (2's comp)"  n_bits=18  bin_pt=16  float_type=Single  exp_bits=8  fraction_bits=24  quantization=Truncate  overflow=Wrap  en=off  latency=1  pipeline=off  dbl_ovrd=off  block_type=convert
  Delay : xbsIndex_r4/Delay  rst=off  infoeditControl=Selection of Reset will increase slice count due to use of real FFs and instead of SRLs  en=off  latency=1  reg_retiming=off  dbl_ovrd=off  block_type=delay
  Delay1 : xbsIndex_r4/Delay  rst=off  infoeditControl=Selection of Reset will increase slice count due to use of real FFs and instead of SRLs  en=off  latency=1  reg_retiming=off  dbl_ovrd=off  block_type=delay
  Display2 : Display
  Gateway Out{1..6,22,24,27} (9 alike) : xbsIndex_r4/Gateway Out  inherit_from_input=off  hdl_port=on  rows=1  columns=1  UseAsDAC=off  DACChannel='1'  interface=None  automatic_assignment=on  address_offset=hex2dec('00')  intf_name=''  intf_description=''  timing_constraint=None  locs_specified=off  LOCs={}  io_standard={}  block_type=gatewayout
  MCode : xbsIndex_r4/MCode  mfname=integration_normalize  explicit_period=off  period=1  inputsTable={'boundInpExpr'=>['','','',''],'inputs'=>['I_int','Q_int','I_int_abs','Q_int_abs']}  outputsTable={'outputs'=>['I_norm','Q_norm','done','bit'],'suppressOut'=>['off','off','off','off']}  enable_stdout=off  enable_debug=off  suppress_output=on  defparams={}  hide_port_list={}  dbl_ovrd=off  block_type=mcode
  Scope1 : Scope  NumInputPorts=4
  Scope11 : Scope  NumInputPorts=4
  I_norm : Outport
  Q_norm : Outport  Port=2
  done : Outport  Port=3
  bit : Outport  Port=4
  wires:
  Gateway Out5/1 -> Scope11/4
  Gateway Out6/1 -> Scope11/3
  Gateway Out3/1 -> Scope1/3
  Gateway Out4/1 -> Scope1/1
  Gateway Out2/1 -> Scope1/4
  Gateway Out1/1 -> Scope1/2
  Convert9/1 -> Gateway Out2/1, I_norm/1
  Convert4/1 -> Gateway Out1/1, Q_norm/1
  MCode/1 -> Gateway Out22/1, Convert9/1, Gateway Out3/1
  Delay/1 -> MCode/1, Gateway Out24/1
  Gateway Out27/1 -> Display2/1
  Gateway Out24/1 -> Scope11/1
  MCode/2 -> Convert4/1, Gateway Out4/1, Gateway Out5/1
  I/1 -> Delay/1, Absolute/1
  MCode/4 -> Gateway Out27/1, bit/1
  Absolute/1 -> MCode/3
  Q/1 -> Absolute1/1, Delay1/1
  Delay1/1 -> MCode/2, Gateway Out6/1
  Gateway Out22/1 -> Scope11/2
  Absolute1/1 -> MCode/4
  MCode/3 -> done/1

== system exampleModel_bus_axi_lcls2/example/dsp/Cav1/IQ_integration2/IQ_latch_normalize1/Subsystem4 ==
  d : Inport
  reset : Inport  Port=2
  Latch : Inport  Port=3
  Register11 : xbsIndex_r4/Register  init=0  rst=on  en=on  dbl_ovrd=off  block_type=register
  posedge_pulse : Subsystem
  q : Outport
  wires:
  reset/1 -> Register11/2
  Latch/1 -> posedge_pulse/1(In1)
  posedge_pulse/1(Out1) -> Register11/3
  Register11/1 -> q/1
  d/1 -> Register11/1

== system exampleModel_bus_axi_lcls2/example/dsp/Cav1/IQ_integration2/IQ_latch_normalize1/Subsystem5 ==
  d : Inport
  reset : Inport  Port=2
  Latch : Inport  Port=3
  Register11 : xbsIndex_r4/Register  init=0  rst=on  en=on  dbl_ovrd=off  block_type=register
  posedge_pulse : Subsystem
  q : Outport
  wires:
  d/1 -> Register11/1
  Register11/1 -> q/1
  posedge_pulse/1(Out1) -> Register11/3
  Latch/1 -> posedge_pulse/1(In1)
  reset/1 -> Register11/2

== system exampleModel_bus_axi_lcls2/example/dsp/Cav1/c1p1_PA_conversion/Subsystem1/posedge_pulse ==
  In1 : Inport
  Inverter1 : xbsIndex_r4/Inverter  en=off  latency=1  dbl_ovrd=off  block_type=inv
  Logical : xbsIndex_r4/Logical  logical_function=AND  inputs=2  en=off  latency=1  precision=Full  arith_type=Unsigned  n_bits=16  bin_pt=0  align_bp=on  dbl_ovrd=off  block_type=logical
  Out1 : Outport
  wires:
  In1/1 -> Logical/1, Inverter1/1
  Logical/1 -> Out1/1
  Inverter1/1 -> Logical/2

== system exampleModel_bus_axi_lcls2/example/dsp/Cav1/c1p1_PA_conversion/Subsystem2/posedge_pulse ==
  In1 : Inport
  Inverter1 : xbsIndex_r4/Inverter  en=off  latency=1  dbl_ovrd=off  block_type=inv
  Logical : xbsIndex_r4/Logical  logical_function=AND  inputs=2  en=off  latency=1  precision=Full  arith_type=Unsigned  n_bits=16  bin_pt=0  align_bp=on  dbl_ovrd=off  block_type=logical
  Out1 : Outport
  wires:
  In1/1 -> Logical/1, Inverter1/1
  Logical/1 -> Out1/1
  Inverter1/1 -> Logical/2

== system exampleModel_bus_axi_lcls2/example/dsp/Cav1/c1p1_PA_conversion/Subsystem3/posedge_pulse ==
  In1 : Inport
  Inverter1 : xbsIndex_r4/Inverter  en=off  latency=1  dbl_ovrd=off  block_type=inv
  Logical : xbsIndex_r4/Logical  logical_function=AND  inputs=2  en=off  latency=1  precision=Full  arith_type=Unsigned  n_bits=16  bin_pt=0  align_bp=on  dbl_ovrd=off  block_type=logical
  Out1 : Outport
  wires:
  Inverter1/1 -> Logical/2
  Logical/1 -> Out1/1
  In1/1 -> Inverter1/1, Logical/1

== system exampleModel_bus_axi_lcls2/example/dsp/Cav1/c1p1_PA_conversion/Subsystem4/posedge_pulse ==
  In1 : Inport
  Inverter1 : xbsIndex_r4/Inverter  en=off  latency=1  dbl_ovrd=off  block_type=inv
  Logical : xbsIndex_r4/Logical  logical_function=AND  inputs=2  en=off  latency=1  precision=Full  arith_type=Unsigned  n_bits=16  bin_pt=0  align_bp=on  dbl_ovrd=off  block_type=logical
  Out1 : Outport
  wires:
  Inverter1/1 -> Logical/2
  Logical/1 -> Out1/1
  In1/1 -> Inverter1/1, Logical/1

== system exampleModel_bus_axi_lcls2/example/dsp/Cav1/c1p1_PA_conversion1/Subsystem1/posedge_pulse ==
  In1 : Inport
  Inverter1 : xbsIndex_r4/Inverter  en=off  latency=1  dbl_ovrd=off  block_type=inv
  Logical : xbsIndex_r4/Logical  logical_function=AND  inputs=2  en=off  latency=1  precision=Full  arith_type=Unsigned  n_bits=16  bin_pt=0  align_bp=on  dbl_ovrd=off  block_type=logical
  Out1 : Outport
  wires:
  In1/1 -> Logical/1, Inverter1/1
  Logical/1 -> Out1/1
  Inverter1/1 -> Logical/2

== system exampleModel_bus_axi_lcls2/example/dsp/Cav1/c1p1_PA_conversion1/Subsystem2/posedge_pulse ==
  In1 : Inport
  Inverter1 : xbsIndex_r4/Inverter  en=off  latency=1  dbl_ovrd=off  block_type=inv
  Logical : xbsIndex_r4/Logical  logical_function=AND  inputs=2  en=off  latency=1  precision=Full  arith_type=Unsigned  n_bits=16  bin_pt=0  align_bp=on  dbl_ovrd=off  block_type=logical
  Out1 : Outport
  wires:
  In1/1 -> Logical/1, Inverter1/1
  Logical/1 -> Out1/1
  Inverter1/1 -> Logical/2

== system exampleModel_bus_axi_lcls2/example/dsp/Cav1/c1p1_PA_conversion1/Subsystem3/posedge_pulse ==
  In1 : Inport
  Inverter1 : xbsIndex_r4/Inverter  en=off  latency=1  dbl_ovrd=off  block_type=inv
  Logical : xbsIndex_r4/Logical  logical_function=AND  inputs=2  en=off  latency=1  precision=Full  arith_type=Unsigned  n_bits=16  bin_pt=0  align_bp=on  dbl_ovrd=off  block_type=logical
  Out1 : Outport
  wires:
  Inverter1/1 -> Logical/2
  Logical/1 -> Out1/1
  In1/1 -> Inverter1/1, Logical/1

== system exampleModel_bus_axi_lcls2/example/dsp/Cav1/c1p1_PA_conversion1/Subsystem4/posedge_pulse ==
  In1 : Inport
  Inverter1 : xbsIndex_r4/Inverter  en=off  latency=1  dbl_ovrd=off  block_type=inv
  Logical : xbsIndex_r4/Logical  logical_function=AND  inputs=2  en=off  latency=1  precision=Full  arith_type=Unsigned  n_bits=16  bin_pt=0  align_bp=on  dbl_ovrd=off  block_type=logical
  Out1 : Outport
  wires:
  Inverter1/1 -> Logical/2
  Logical/1 -> Out1/1
  In1/1 -> Inverter1/1, Logical/1
